simulink library "INT_CoETS_StTrqLimCalc"  (R2016b)
settings: Solver=VariableStepAuto  StartTime=0.0  StopTime=10.0  RelTol=1e-3
settings Model: Creator=Administrator  LastModifiedBy=Administrator

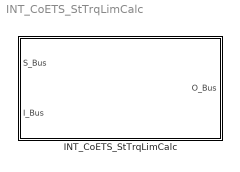
== system INT_CoETS_StTrqLimCalc ==
  INT_CoETS_StTrqLimCalc : Subsystem

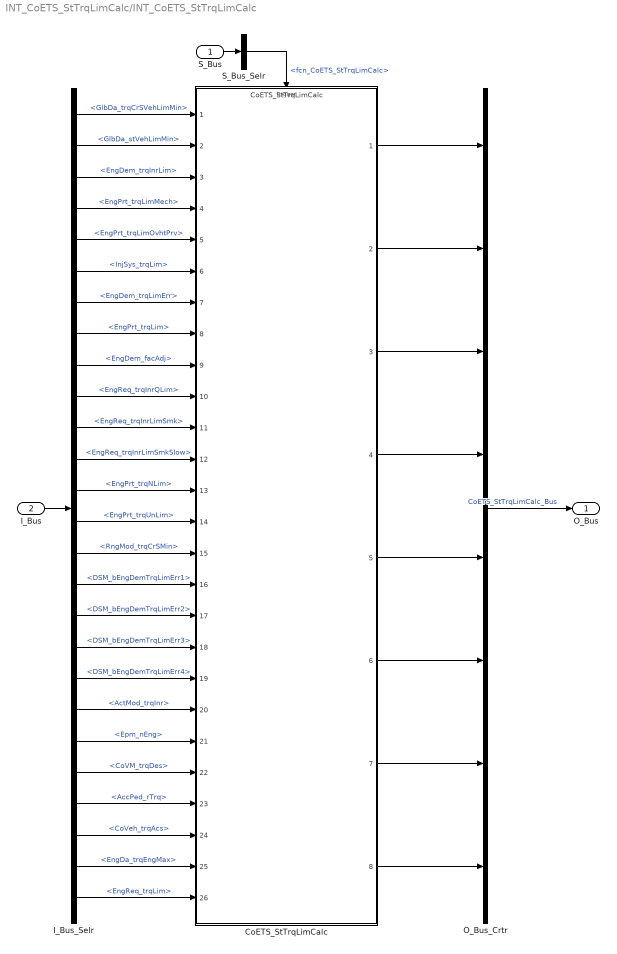
== system INT_CoETS_StTrqLimCalc/INT_CoETS_StTrqLimCalc ==
  S_Bus : Inport
  I_Bus : Inport  Port=2
  CoETS_StTrqLimCalc : ModelReference  ModelNameDialog=CoETS_StTrqLimCalc  SimulationMode=Normal  ModelReferenceVersion=1.3  TriggerPortName=function  TriggerPortTriggerType=function-call  TriggerPortStatesWhenEnabling=held
  I_Bus_Selr : BusSelector  OutputSignals=GlbDa_trqCrSVehLimMin,GlbDa_stVehLimMin,EngDem_trqInrLim,EngPrt_trqLimMech,EngPrt_trqLimOvhtPrv,InjSys_trqLim,EngDem_trqLimErr,EngPrt_trqLim,EngDem_facAdj,EngReq_trqInrQLim,EngReq_trqInrLimSmk,EngReq_trqInrLimSmkSlow,EngPrt_trqNLim,EngPrt_trqUnLim,RngMod_trqCrSMin,DSM_bEngDemTrqLimErr1,DSM_bEngDemTrqLimErr2,DSM_bEngDemTrqLimErr3,DSM_bEngDemTrqLimErr4,ActMod_trqInr,Epm_nEng,CoVM_trqDes,AccPed_rTrq,CoVeh_trqAcs,EngDa_trqEngMax,EngReq_trqLim
  O_Bus_Crtr : BusCreator  Inputs=8
  S_Bus_Selr : BusSelector  OutputSignals=fcn_CoETS_StTrqLimCalc
  O_Bus : Outport
  wires:
  S_Bus_Selr/1 -> CoETS_StTrqLimCalc/Trigger  "<fcn_CoETS_StTrqLimCalc>"
  S_Bus/1 -> S_Bus_Selr/1
  I_Bus/1 -> I_Bus_Selr/1
  I_Bus_Selr/1 -> CoETS_StTrqLimCalc/1  "<GlbDa_trqCrSVehLimMin>"
  I_Bus_Selr/2 -> CoETS_StTrqLimCalc/2  "<GlbDa_stVehLimMin>"
  I_Bus_Selr/3 -> CoETS_StTrqLimCalc/3  "<EngDem_trqInrLim>"
  I_Bus_Selr/4 -> CoETS_StTrqLimCalc/4  "<EngPrt_trqLimMech>"
  I_Bus_Selr/5 -> CoETS_StTrqLimCalc/5  "<EngPrt_trqLimOvhtPrv>"
  I_Bus_Selr/6 -> CoETS_StTrqLimCalc/6  "<InjSys_trqLim>"
  I_Bus_Selr/7 -> CoETS_StTrqLimCalc/7  "<EngDem_trqLimErr>"
  I_Bus_Selr/8 -> CoETS_StTrqLimCalc/8  "<EngPrt_trqLim>"
  I_Bus_Selr/9 -> CoETS_StTrqLimCalc/9  "<EngDem_facAdj>"
  I_Bus_Selr/10 -> CoETS_StTrqLimCalc/10  "<EngReq_trqInrQLim>"
  I_Bus_Selr/11 -> CoETS_StTrqLimCalc/11  "<EngReq_trqInrLimSmk>"
  I_Bus_Selr/12 -> CoETS_StTrqLimCalc/12  "<EngReq_trqInrLimSmkSlow>"
  I_Bus_Selr/13 -> CoETS_StTrqLimCalc/13  "<EngPrt_trqNLim>"
  I_Bus_Selr/14 -> CoETS_StTrqLimCalc/14  "<EngPrt_trqUnLim>"
  I_Bus_Selr/15 -> CoETS_StTrqLimCalc/15  "<RngMod_trqCrSMin>"
  I_Bus_Selr/16 -> CoETS_StTrqLimCalc/16  "<DSM_bEngDemTrqLimErr1>"
  I_Bus_Selr/17 -> CoETS_StTrqLimCalc/17  "<DSM_bEngDemTrqLimErr2>"
  I_Bus_Selr/18 -> CoETS_StTrqLimCalc/18  "<DSM_bEngDemTrqLimErr3>"
  I_Bus_Selr/19 -> CoETS_StTrqLimCalc/19  "<DSM_bEngDemTrqLimErr4>"
  I_Bus_Selr/20 -> CoETS_StTrqLimCalc/20  "<ActMod_trqInr>"
  I_Bus_Selr/21 -> CoETS_StTrqLimCalc/21  "<Epm_nEng>"
  I_Bus_Selr/22 -> CoETS_StTrqLimCalc/22  "<CoVM_trqDes>"
  I_Bus_Selr/23 -> CoETS_StTrqLimCalc/23  "<AccPed_rTrq>"
  I_Bus_Selr/24 -> CoETS_StTrqLimCalc/24  "<CoVeh_trqAcs>"
  I_Bus_Selr/25 -> CoETS_StTrqLimCalc/25  "<EngDa_trqEngMax>"
  I_Bus_Selr/26 -> CoETS_StTrqLimCalc/26  "<EngReq_trqLim>"
  O_Bus_Crtr/1 -> O_Bus/1  "CoETS_StTrqLimCalc_Bus"
  CoETS_StTrqLimCalc/1 -> O_Bus_Crtr/1
  CoETS_StTrqLimCalc/2 -> O_Bus_Crtr/2
  CoETS_StTrqLimCalc/3 -> O_Bus_Crtr/3
  CoETS_StTrqLimCalc/4 -> O_Bus_Crtr/4
  CoETS_StTrqLimCalc/5 -> O_Bus_Crtr/5
  CoETS_StTrqLimCalc/6 -> O_Bus_Crtr/6
  CoETS_StTrqLimCalc/7 -> O_Bus_Crtr/7
  CoETS_StTrqLimCalc/8 -> O_Bus_Crtr/8
